simulink model "rudder_Subsystem"  (Simulink 7.8)
settings: Solver=FixedStepDiscrete  SolverMode=SingleTasking  StartTime=0.0  StopTime=10.0  FixedStep=0.01  RelTol=1e-3
InitFcn:
  | clear all
  | common
  | Busses
values from neighbouring files (symbols this model uses):
  T_step = 0.01    [common.m]
undefined symbols (not defined in the file or in its folder): ANmax, CalculateRudderAngle, DataEEInitAndClear, Init_onlyOnce, Init_Reset, initCalibrationRange, InitRudderCalibrationRange, OC1max, RudderCalibrate, RudderEcanInit, RudderSubsystemInit, SendAndReceiveEcan
libraries: dsPICdrivers x17, simulink x4, ecan_dspic x1
settings Model: Creator=bwmairs  LastModifiedBy=Bryant
settings OptimizationCC: InlineParams=on  InlineInvariantSignals=on  InitFltsAndDblsToZero=on  EfficientFloat2IntCast=on
settings DebuggingCC: ReadBeforeWriteMsg=DisableAll  WriteAfterWriteMsg=DisableAll  WriteAfterReadMsg=DisableAll  UnderspecifiedInitializationDetection=Simplified  ParameterOverflowMsg=warning  FcnCallInpInsideContextMsg=Use local settings  UniqueDataStoreMsg=error
settings HardwareCC: ProdBitPerInt=16  ProdBitPerPointer=16  ProdIntDivRoundTo=Zero  ProdEndianess=LittleEndian  ProdWordSize=16  ProdHWDeviceType=16-bit Generic
settings ModelReferenceCC: ModelReferenceNumInstancesAllowed=Single
settings SFSimCC: SimParseCustomCode=off
settings RTWCC: SystemTargetFile=dspic.tlc  GenCodeOnly=on  MakeCommand=make_CreateMPLAB  TemplateMakefile=dspic_pic30_gcc.tmf  PostCodeGenCommand=dsPIC_Compile()  Description=Embedded Target for Microchip dsPIC (real-time)  ProcessScript=dspic_make_rtw_hook  RTWCompilerOptimization=On
settings RTWCC: CustomInclude=|
  | ../../../mavlink/seaslug/sealion
  | ../../../mavlink/seaslug/
  | clib
  | ../basic_model/clib
settings RTWCC: CustomSource=|
  | clib/ecanRudder.c
  | clib/traps.c
  | clib/Nvram.c
  | 
  | ../basic_model/clib/nmea2000.c
  | ../basic_model/clib/DEE.c
  | ../basic_model/clib/DEES.s
  | ../basic_model/clib/MavlinkMessageScheduler.c
  | 
  | ../../../ECAN_dspic/CircularBuffer.c
  | ../../../ECAN_dspic/ecanFunctions.c
settings STFCustomTargetCC: TargetFunctionLibrary=C89/C90 (ANSI)  IncludeMdlTerminateFcn=off  SupportNonInlinedSFcns=off  SystemTargetFile=dspic.tlc
settings ERTTargetCC: TargetFunctionLibrary=C89/C90 (ANSI)  MultiwordLength=2048  ParMdlRefBuildCompliant=off  CompOptLevelCompliant=off  ConcurrentExecutionCompliant=off  IncludeMdlTerminateFcn=off  GeneratePreprocessorConditionals=Disable all  CombineOutputUpdateFcns=off  ERTFirstTimeCompliant=off  ERTCustomFileBanners=off  SupportContinuousTime=on  ModelStepFunctionPrototypeControlCompliant=off  CPPClassGenCompliant=off  ExtModeMexFile=ext_serial_win32_comm  InlinedParameterPlacement=NonHierarchical  ERTSrcFileBannerTemplate=dsPIC_code_template.cgt  ERTHdrFileBannerTemplate=dsPIC_code_template.cgt  ERTDataSrcFileTemplate=dsPIC_code_template.cgt  ERTDataHdrFileTemplate=dsPIC_code_template.cgt  ERTCustomFileTemplate=dsPIC_main.tlc  ConvertIfToSwitch=off  SuppressUnreachableDefaultCases=off
settings CustomProperty: DataType=string  Value=C:\PROGRA~1\MATLAB\R2011b\bin\win64\gmake

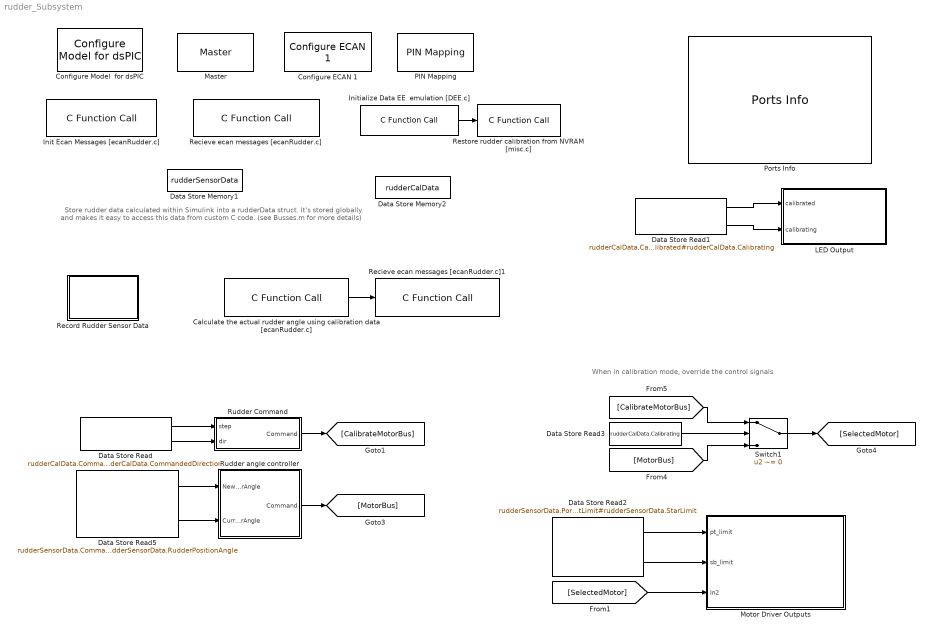
== system rudder_Subsystem ==
  note: When in calibration mode, override the
      | control signals
  note: Store rudder data calculated within Simulink into a rudderData struct.
      | It's stored globally and makes it easy to access this data from custom
      | C code. (see Busses.m for more details)
  Calculate the actual rudder angle using calibration data [ecanRudder.c] : dsPICdrivers/OTHERS/C Function Call  Tag=dsPIC_dsPIC_CFunctionCall  FctUpdate=Output Function  fctName=CalculateRudderAngle  INPUT_SIZE=1  INPUT1=--  INPUT2=--  INPUT3=--  OUTPUT_SIZE=1  OUTPUT1=--  SampleTime=T_step  InputType=[ ]  OutputType=[ ]  FctDeclaration=extern void CalculateRudderAngle();  FctCall=CalculateRudderAngle();  OrderingInOutPopup=Output  FctStart=None  FctStart_Name=Init_onlyOnce  FctStart_Declaration=inline extern void Init_onlyOnce();  FctStart_Call=Init_onlyOnce();  FctInit=None  FctInit_Name=Init_Reset  FctInit_Declaration=inline extern void Init_Reset();  FctInit_Call=Init_Reset();  PinDigitalInput=[]  PinDigitalOutput=[]  AnalogueInput=[]
  Configure ECAN 1 : ecan_dspic/Configure ECAN 1  frame_setting=on  mode=Normal  dma_rx_chan=2  dma_tx_chan=0  baud=250000  ps1=8  pd=5  ps2=6  sjw=4  tq=20  triple_sample=on  dma_buf_size=4 buffers  rx_bufs=[1]  tx_bufs=[0]  buf_0_tx_pri=Highest  buf_0_rte=No  buf_1_tx_pri=Highest  buf_1_rte=No  buf_2_tx_pri=Lowest  buf_2_rte=No  buf_3_tx_pri=Lowest  buf_3_rte=No  buf_4_tx_pri=Lowest  buf_4_rte=No  buf_5_tx_pri=Lowest  buf_5_rte=No  buf_6_tx_pri=Lowest  buf_6_rte=No  buf_7_tx_pri=Lowest  buf_7_rte=No  mask_0=0  mask_0_mide=Match std or ext  mask_1=0  mask_1_mide=Match std or ext  mask_2=0  mask_2_mide=Match std or ext  filters=[0]  filter_0=0  filter_0_mask=0  filter_0_exide=Match only standard  filter_0_buf=1  filter_1=hex2dec('401')  filter_1_mask=0  filter_1_exide=Match only standard  filter_1_buf=2  filter_2=hex2dec('402')  filter_2_mask=0  filter_2_exide=Match only standard  filter_2_buf=3  filter_3=0  filter_3_mask=0  filter_3_exide=Match only standard  filter_3_buf=0  filter_4=0  filter_4_mask=0  filter_4_exide=Match only standard  filter_4_buf=0  filter_5=0  filter_5_mask=0  filter_5_exide=Match only standard  filter_5_buf=0  filter_6=0  filter_6_mask=0  filter_6_exide=Match only standard  filter_6_buf=0  filter_7=0  filter_7_mask=0  filter_7_exide=Match only standard  filter_7_buf=0  filter_8=0  filter_8_mask=0  filter_8_exide=Match only standard  filter_8_buf=0  filter_9=0  filter_9_mask=<empty>  filter_9_exide=Match only standard  filter_9_buf=0  filter_10=0  filter_10_mask=0  filter_10_exide=Match only standard  filter_10_buf=0  filter_11=0  filter_11_mask=0  filter_11_exide=Match only standard  filter_11_buf=0  filter_12=0  filter_12_mask=0  filter_12_exide=Match only standard  filter_12_buf=0  filter_13=0  filter_13_mask=0  filter_13_exide=Match only standard  filter_13_buf=0  filter_14=0  filter_14_mask=0  filter_14_exide=Match only standard  filter_14_buf=0  filter_15=0  filter_15_mask=0  filter_15_exide=Match only standard  filter_15_buf=0
  Configure Model  for dsPIC : dsPICdrivers/Simulink Configuration/Configure Model  for dsPIC
  Data Store Memory1 : DataStoreMemory  DataStoreName=rudderSensorData  ReadBeforeWriteMsg=warning  WriteAfterWriteMsg=warning  WriteAfterReadMsg=warning  OutDataTypeStr=Bus: RudderVariables
      settings: RTWStateStorageClass=ImportedExtern
  Data Store Memory2 : DataStoreMemory  DataStoreName=rudderCalData  ReadBeforeWriteMsg=warning  WriteAfterWriteMsg=warning  WriteAfterReadMsg=warning  OutDataTypeStr=Bus: RudderCalData
      settings: RTWStateStorageClass=ImportedExtern
  Data Store Read : DataStoreRead  DataStoreName=rudderCalData  SampleTime=T_step  DataStoreElements=rudderCalData.CommandedRun#rudderCalData.CommandedDirection
  Data Store Read1 : DataStoreRead  DataStoreName=rudderCalData  SampleTime=T_step  DataStoreElements=rudderCalData.Calibrated#rudderCalData.Calibrating
  Data Store Read2 : DataStoreRead  DataStoreName=rudderSensorData  SampleTime=T_step  DataStoreElements=rudderSensorData.PortLimit#rudderSensorData.StarLimit
  Data Store Read3 : DataStoreRead  DataStoreName=rudderCalData  SampleTime=T_step  DataStoreElements=rudderCalData.Calibrating
  Data Store Read5 : DataStoreRead  DataStoreName=rudderSensorData  SampleTime=T_step  DataStoreElements=rudderSensorData.CommandedRudderAngle#rudderSensorData.RudderPositionAngle
  Init Ecan Messages [ecanRudder.c] : dsPICdrivers/OTHERS/C Function Call  Tag=dsPIC_dsPIC_CFunctionCall  FctUpdate=None  fctName=RudderEcanInit  INPUT_SIZE=1  INPUT1=--  INPUT2=--  INPUT3=--  OUTPUT_SIZE=-1  OUTPUT1=--  SampleTime=Inf  InputType=[]  OutputType=[]  FctDeclaration=extern void RudderEcanInit();  FctCall=RudderEcanInit();  OrderingInOutPopup=None  FctStart=Start Function (Call once and only once)  FctStart_Name=RudderSubsystemInit  FctStart_Declaration=inline extern void RudderSubsystemInit();  FctStart_Call=RudderSubsystemInit();  FctInit=None  FctInit_Name=RudderEcanInit  FctInit_Declaration=inline extern void RudderEcanInit();  FctInit_Call=RudderEcanInit();  PinDigitalInput=[]  PinDigitalOutput=[]  AnalogueInput=[]
  Initialize Data EE  emulation [DEE.c] : dsPICdrivers/OTHERS/C Function Call  Tag=dsPIC_dsPIC_CFunctionCall  FctUpdate=None  fctName='DataEEInitAndClear'  INPUT_SIZE=1  INPUT1=--  INPUT2=--  INPUT3=--  OUTPUT_SIZE=1  OUTPUT1=--  SampleTime=Inf  InputType=[]  OutputType=[]  FctDeclaration=extern void DataEEInitAndClear();  FctCall=DataEEInitAndClear();  OrderingInOutPopup=Output  FctStart=Start Function (Call once and only once)  FctStart_Name=DataEEInitAndClear  FctStart_Declaration=inline extern void DataEEInitAndClear();  FctStart_Call=DataEEInitAndClear();  FctInit=None  FctInit_Name=Init_Reset  FctInit_Declaration=inline extern void Init_Reset();  FctInit_Call=Init_Reset();  PinDigitalInput=[]  PinDigitalOutput=[]  AnalogueInput=[]
  LED Output : Subsystem
  Master : dsPICdrivers/Master  Tag=dsPIC_MASTER  Priority=1  TimeStepType=Timer1  picType=33fj128MC802  fcy=40008571.4286  Quartz_33f=8e6  PLLActive_33f=on  fcyDesired_33f=40000000  tmr1="[8  50010  -0.00057131]"  tmr1Info="Time Step : 0.01  ;   Error : -0.00057131%  PR1=50010"  tmr2345="[8  0  0  0]"  tmr2345cfg=[-1 -1 -1 -1]  IOautoConf=on  typePort="[ 9   8   0   0  10   0   0   0   0   0   0   0   0   0   0   0   0   9   8   0  22   0   0  23   0  10  10   0  23   0   0   0   0   0   0   0   0   0   0   0   0   0   0   0   0   0   0   0   0   0   0   0   0   0   0   0   0   0   0   0   0   0   0   0   0   0   0   0   0   0   0   0   0   0   0   0   0   0   0   0   0   0   0   0   0   0   0   0   0   0   0   0   0   0   0   0   0   0   0   0   0   0   0   0   0   0   0   0   0   0   0   0 ]"  TRIS="[ 65519  59775  65535  65535  65535  65535  65535 ]"  ADPCFG=9  MasterBusyPort=None  MasterOverloadPort=None  FOSC=Internal Fast RC 7.37Mhz  ClockSwitchMonitor=Both disabled  TempProtection_33f=TEMP_ON  FPBOR=<empty>  PWRT=disable  MCLR=<empty>  ICD=ICS_PGD3  JTAGEN=JTAGEN_OFF  PowerSave=off  OverrideFcy=off  NewFcy=1e6  PR2345="[65535  65535  65535  65535]"
  Motor Driver Outputs : Subsystem
  PIN Mapping : dsPICdrivers/Peripheral MAPPING/PIN Mapping  Tag=dsPIC_PIN_Mapping  in_INT1=Not tied (VSS)  in_INT2=Not tied (VSS)  in_T2CK=Not tied (VSS)  in_T3CK=Not tied (VSS)  in_T4CK=Not tied (VSS)  in_T5CK=Not tied (VSS)  in_IC1=Not tied (VSS)  in_IC2=Not tied (VSS)  in_IC7=Not tied (VSS)  in_IC8=Not tied (VSS)  out_OC1=tied to RP12  out_OC2=Not changed  out_OC3=Not changed  out_OC4=Not changed  in_OCFA=Not tied (VSS)  in_FLTA1=Not tied (VSS)  in_FLTA2=Not tied (VSS)  in_QEA1=Not tied (VSS)  in_QEB1=Not tied (VSS)  in_INDX1=Not tied (VSS)  out_UPDN1=Not changed  out_UPDN2=Not changed  in_QEA2=Not tied (VSS)  in_QEB2=Not tied (VSS)  in_INDX2=Not tied (VSS)  in_U1RX=Not tied (VSS)  out_U1TX=Not changed  in_U1CTS=Not tied (VSS)  out_U1RTS=Not changed  in_U2RX=Not tied (VSS)  out_U2TX=Not changed  in_U2CTS=Not tied (VSS)  out_U2RTS=Not changed  in_SDI1=Not tied (VSS)  out_SDO1=Not changed  in_SCK1=Not tied (VSS)  out_SCK1OUT=Not changed  in_SS1=Not tied (VSS)  out_SS1OUT=Not changed  in_SDI2=Not tied (VSS)  out_SDO2=Not changed  in_SCK2=Not tied (VSS)  out_SCK2OUT=Not changed  in_SS2=Not tied (VSS)  out_SS2OUT=Not changed  in_C1RX=tied to RP4  out_C1TX=tied to RP7  out_C1OUT=Not changed  out_C2OUT=Not changed
  Ports Info : dsPICdrivers/Ports Info  Tag=dsPIC_PortInfo
  Recieve ecan messages [ecanRudder.c] : dsPICdrivers/OTHERS/C Function Call  Tag=dsPIC_dsPIC_CFunctionCall  FctUpdate=Output Function  fctName=SendAndReceiveEcan  INPUT_SIZE=1  INPUT1=--  INPUT2=--  INPUT3=--  OUTPUT_SIZE=1  OUTPUT1=--  SampleTime=.01  InputType=[ ]  OutputType=[ ]  FctDeclaration=extern void SendAndReceiveEcan();  FctCall=SendAndReceiveEcan();  OrderingInOutPopup=None  FctStart=None  FctStart_Name=Init_onlyOnce  FctStart_Declaration=inline extern void Init_onlyOnce();  FctStart_Call=Init_onlyOnce();  FctInit=None  FctInit_Name=Init_Reset  FctInit_Declaration=inline extern void Init_Reset();  FctInit_Call=Init_Reset();  PinDigitalInput=[]  PinDigitalOutput=[]  AnalogueInput=[]
  Recieve ecan messages [ecanRudder.c]1 : dsPICdrivers/OTHERS/C Function Call  Tag=dsPIC_dsPIC_CFunctionCall  FctUpdate=Output Function  fctName=RudderCalibrate  INPUT_SIZE=1  INPUT1=--  INPUT2=--  INPUT3=--  OUTPUT_SIZE=1  OUTPUT1=--  SampleTime=T_step  InputType=[ ]  OutputType=[ ]  FctDeclaration=extern void RudderCalibrate();  FctCall=RudderCalibrate();  OrderingInOutPopup=Input  FctStart=None  FctStart_Name=Init_onlyOnce  FctStart_Declaration=inline extern void Init_onlyOnce();  FctStart_Call=Init_onlyOnce();  FctInit=None  FctInit_Name=Init_Reset  FctInit_Declaration=inline extern void Init_Reset();  FctInit_Call=Init_Reset();  PinDigitalInput=[]  PinDigitalOutput=[]  AnalogueInput=[]
  Record Rudder Sensor Data : Subsystem
  Restore rudder calibration from NVRAM [misc.c] : dsPICdrivers/OTHERS/C Function Call  Tag=dsPIC_dsPIC_CFunctionCall  FctUpdate=None  fctName='initCalibrationRange'  INPUT_SIZE=1  INPUT1=--  INPUT2=--  INPUT3=--  OUTPUT_SIZE=1  OUTPUT1=--  SampleTime=Inf  InputType=[]  OutputType=[]  FctDeclaration=extern void initCalibrationRange();  FctCall=initCalibrationRange();  OrderingInOutPopup=Input  FctStart=Start Function (Call once and only once)  FctStart_Name=InitRudderCalibrationRange  FctStart_Declaration=inline extern void InitRudderCalibrationRange();  FctStart_Call=InitRudderCalibrationRange();  FctInit=None  FctInit_Name=Init_Reset  FctInit_Declaration=inline extern void Init_Reset();  FctInit_Call=Init_Reset();  PinDigitalInput=[]  PinDigitalOutput=[]  AnalogueInput=[]
  Rudder Command : Subsystem
  Rudder angle controller : Subsystem
  Switch1 : Switch  Criteria=u2 ~= 0
  wires:
  Data Store Read/1 -> Rudder Command/1(step)
  Data Store Read/2 -> Rudder Command/2(dir)
  Rudder Command/1(Command) -> [CalibrateMotorBus]
  [SelectedMotor] -> Motor Driver Outputs/3(In2)
  Rudder angle controller/1(Command) -> [MotorBus]
  [CalibrateMotorBus] -> Switch1/1
  [MotorBus] -> Switch1/3
  Switch1/1 -> [SelectedMotor]
  Data Store Read5/2 -> Rudder angle controller/2(CurrentRudderAngle)
  Data Store Read5/1 -> Rudder angle controller/1(NewRudderAngle)
  Initialize Data EE  emulation [DEE.c]/1 -> Restore rudder calibration from NVRAM [misc.c]/1
  Calculate the actual rudder angle using calibration data [ecanRudder.c]/1 -> Recieve ecan messages [ecanRudder.c]1/1
  Data Store Read1/1 -> LED Output/1(calibrated)
  Data Store Read1/2 -> LED Output/2(calibrating)
  Data Store Read2/1 -> Motor Driver Outputs/1(pt_limit)
  Data Store Read2/2 -> Motor Driver Outputs/2(sb_limit)
  Data Store Read3/1 -> Switch1/2

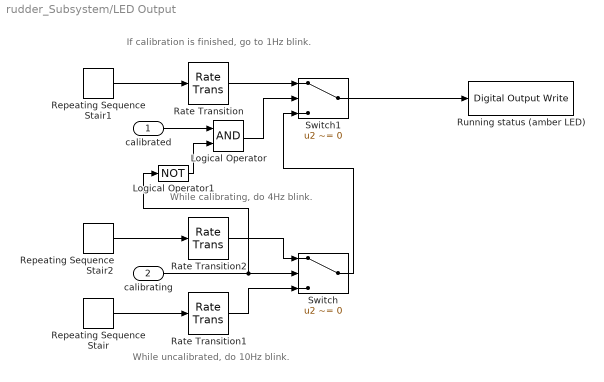
== system rudder_Subsystem/LED Output ==
  note: If calibration is finished, go to 1Hz blink.
  note: While calibrating, do 4Hz blink.
  note: While uncalibrated, do 10Hz blink.
  calibrated : Inport
  calibrating : Inport  Port=2
  Logical Operator : Logic  AllPortsSameDT=off  OutDataTypeStr=boolean
  Logical Operator1 : Logic  Operator=NOT  AllPortsSameDT=off  OutDataTypeStr=boolean
  Rate Transition : RateTransition
  Rate Transition1 : RateTransition
  Rate Transition2 : RateTransition
  Repeating Sequence Stair : simulink/Sources/Repeating Sequence Stair  OutValues=[1 0]  tsamp=.1  OutMin=[]  OutMax=[]  OutDataTypeStr=fixdt('boolean')  OutputDataTypeScalingMode=Specify via dialog  OutDataType=fixdt('boolean')  ConRadixGroup=Best Precision: Vector-wise  OutScaling=[]
  Repeating Sequence Stair1 : simulink/Sources/Repeating Sequence Stair  OutValues=[1 0]  tsamp=1  OutMin=[]  OutMax=[]  OutDataTypeStr=fixdt('boolean')  OutputDataTypeScalingMode=Specify via dialog  OutDataType=fixdt('boolean')  ConRadixGroup=Best Precision: Vector-wise  OutScaling=[]
  Repeating Sequence Stair2 : simulink/Sources/Repeating Sequence Stair  OutValues=[1 0]  tsamp=.25  OutMin=[]  OutMax=[]  OutDataTypeStr=fixdt('boolean')  OutputDataTypeScalingMode=Specify via dialog  OutDataType=fixdt('boolean')  ConRadixGroup=Best Precision: Vector-wise  OutScaling=[]
  Running status (amber LED) : dsPICdrivers/Digital I//O/Digital Output Write  Tag=dsPIC_Digital_Output  Priority=5  PORT=A  Pin=[4]  Simultaneous=off  OrderingInOutPopup=None
  Switch : Switch  Criteria=u2 ~= 0
  Switch1 : Switch  Criteria=u2 ~= 0
  wires:
  Repeating Sequence Stair/1 -> Rate Transition1/1
  Rate Transition1/1 -> Switch/3
  calibrating/1 -> Switch/2, Logical Operator1/1
  Repeating Sequence Stair1/1 -> Rate Transition/1
  Rate Transition/1 -> Switch1/1
  Repeating Sequence Stair2/1 -> Rate Transition2/1
  Rate Transition2/1 -> Switch/1
  Switch1/1 -> Running status (amber LED)/1
  Switch/1 -> Switch1/3
  calibrated/1 -> Logical Operator/1
  Logical Operator/1 -> Switch1/2
  Logical Operator1/1 -> Logical Operator/2

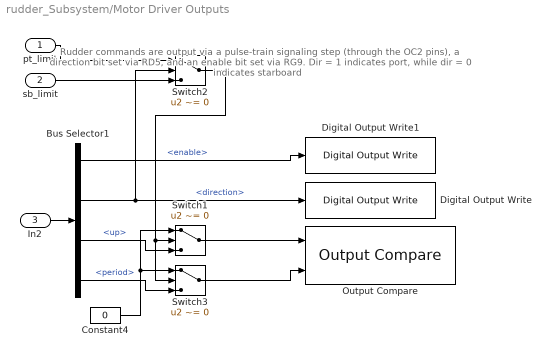
== system rudder_Subsystem/Motor Driver Outputs ==
  note: Rudder commands are output via a pulse-train signaling step (through the OC2 pins),
      | a direction bit set via RD5, and an enable bit set via RG9. Dir = 1 indicates port, while
      | dir = 0 indicates starboard
  pt_limit : Inport
  sb_limit : Inport  Port=2
  In2 : Inport  Port=3
  Bus Selector1 : BusSelector  OutputSignals=enable,direction,up,period
  Constant4 : Constant  Value=0  OutDataTypeStr=uint16
  Digital Output Write : dsPICdrivers/Digital I//O/Digital Output Write  Tag=dsPIC_Digital_Output  Priority=5  PORT=B  Pin=[9]  Simultaneous=off  OrderingInOutPopup=None
  Digital Output Write1 : dsPICdrivers/Digital I//O/Digital Output Write  Tag=dsPIC_Digital_Output  Priority=5  PORT=B  Pin=[10]  Simultaneous=off  OrderingInOutPopup=None
  Output Compare : dsPICdrivers/Peripheral I//O/Output Compare  Tag=dsPIC_PWM_out  Priority=5  IntPriority=3  CHANNEL=[1]  Channel_UP_Down_Periode=[5]  MaxChannel=[0.01]  MaxName=' OC1max '  Precision=[15.6099]  Timer=[2]  Status=OK  SafeMarge=[0]  PortLetter=[66]  PortNumber=[12]  MaxValues=[50010]
  Switch1 : Switch  Criteria=u2 ~= 0  Threshold=1  OutDataTypeStr=Inherit: Inherit via back propagation
  Switch2 : Switch  Criteria=u2 ~= 0  Threshold=1  OutDataTypeStr=Inherit: Inherit via back propagation
  Switch3 : Switch  Criteria=u2 ~= 0  Threshold=1  OutDataTypeStr=Inherit: Inherit via back propagation
  wires:
  Bus Selector1/1 -> Digital Output Write1/1  "<enable>"
  Switch2/1 -> Switch1/2, Switch3/2
  Constant4/1 -> Switch1/1, Switch3/1
  Bus Selector1/4 -> Switch3/3  "<period>"
  Bus Selector1/3 -> Switch1/3  "<up>"
  Switch1/1 -> Output Compare/1
  Switch3/1 -> Output Compare/2
  Bus Selector1/2 -> Digital Output Write/1, Switch2/2  "<direction>"
  pt_limit/1 -> Switch2/1
  In2/1 -> Bus Selector1/1
  sb_limit/1 -> Switch2/3

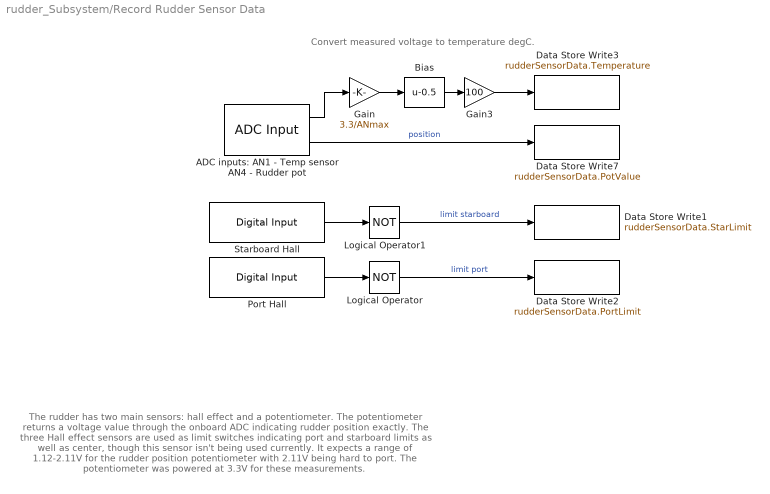
== system rudder_Subsystem/Record Rudder Sensor Data ==
  note: The rudder has two main sensors: hall effect and a potentiometer. The
      | potentiometer returns a voltage value through the onboard ADC indicating
      | rudder position exactly. The three Hall effect sensors are used as limit switches
      | indicating port and starboard limits as well as center, though this sensor isn't
      | being used currently.
      |
      | It expects a range of 1.12-2.11V for the rudder position potentiometer with
      | 2.11V being hard to port. The potentiometer was powered at 3.3V for these
      | measurements.
  note: Convert measured voltage to temperature degC.
  ADC inputs: AN1 - Temp sensor AN4 - Rudder pot : dsPICdrivers/Peripheral I//O/ADC Input  Tag=dsPIC_ADC  Priority=5  ADC_TYPE=12 bits  ADC_MODE=Continuous sampling & get last channel value  NbrSampleStep=1  VoltRefpopup="AVdd  -  AVss"  OutFormatBitspopup=0000 dddd dddd dddd : Integer  InterruptPriority=6  ANCHANNELS=[4 1]  MaxName=ANmax = 4095  Rin=0  ADCS=53  SAMC=1  Temperature=25  DMAChannel=1  SampleTime=T_step  Status="OK  |  Tsmp=6.749e-007 |  T/Channel=1.012e-005 |  Tall=2.025e-005"  SSRC=auto convert
  Bias : Bias  Bias=-0.5
  Data Store Write1 : DataStoreWrite  DataStoreName=rudderSensorData  DataStoreElements=rudderSensorData.StarLimit
  Data Store Write2 : DataStoreWrite  DataStoreName=rudderSensorData  DataStoreElements=rudderSensorData.PortLimit
  Data Store Write3 : DataStoreWrite  DataStoreName=rudderSensorData  DataStoreElements=rudderSensorData.Temperature
  Data Store Write7 : DataStoreWrite  DataStoreName=rudderSensorData  DataStoreElements=rudderSensorData.PotValue
  Gain : Gain  Gain=3.3/ANmax  ParamDataTypeStr=single  OutDataTypeStr=single  RndMeth=Simplest
  Gain3 : Gain  Gain=100  ParamDataTypeStr=single  OutDataTypeStr=single  RndMeth=Simplest
  Logical Operator : Logic  Operator=NOT  Inputs=1  AllPortsSameDT=off  OutDataTypeStr=boolean
  Logical Operator1 : Logic  Operator=NOT  Inputs=1  AllPortsSameDT=off  OutDataTypeStr=boolean
  Port Hall : dsPICdrivers/Digital I//O/Digital Input  Tag=dsPIC_Digital_Input  PORT=A  Pin=[0]  SampleTime=T_step  OrderingInOutPopup=None
  Starboard Hall : dsPICdrivers/Digital I//O/Digital Input  Tag=dsPIC_Digital_Input  PORT=B  Pin=[1]  SampleTime=T_step  OrderingInOutPopup=None
  wires:
  Logical Operator1/1 -> Data Store Write1/1  "limit starboard"
  Logical Operator/1 -> Data Store Write2/1  "limit port"
  Port Hall/1 -> Logical Operator/1
  Starboard Hall/1 -> Logical Operator1/1
  ADC inputs: AN1 - Temp sensor AN4 - Rudder pot/2 -> Data Store Write7/1  "position"
  ADC inputs: AN1 - Temp sensor AN4 - Rudder pot/1 -> Gain/1
  Gain/1 -> Bias/1
  Bias/1 -> Gain3/1
  Gain3/1 -> Data Store Write3/1

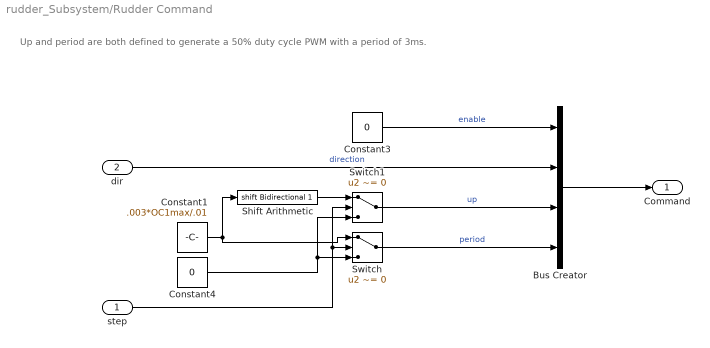
== system rudder_Subsystem/Rudder Command ==
  note: Up and period are both defined to generate a 50% duty cycle PWM with
      | a period of 3ms.
  step : Inport
  dir : Inport  Port=2
  Bus Creator : BusCreator
  Constant1 : Constant  Value=.003*OC1max/.01  OutDataTypeStr=uint16
  Constant3 : Constant  Value=0  OutDataTypeStr=boolean
  Constant4 : Constant  Value=0  OutDataTypeStr=uint16
  Shift Arithmetic : ArithShift  BitShiftNumber=1
  Switch : Switch  Criteria=u2 ~= 0
  Switch1 : Switch  Criteria=u2 ~= 0
  Command : Outport
  wires:
  step/1 -> Switch1/2, Switch/2
  Constant4/1 -> Switch1/3, Switch/3
  Switch1/1 -> Bus Creator/3  "up"
  Switch/1 -> Bus Creator/4  "period"
  Shift Arithmetic/1 -> Switch1/1
  Constant1/1 -> Switch/1, Shift Arithmetic/1
  Constant3/1 -> Bus Creator/1  "enable"
  Bus Creator/1 -> Command/1
  dir/1 -> Bus Creator/2  "direction"

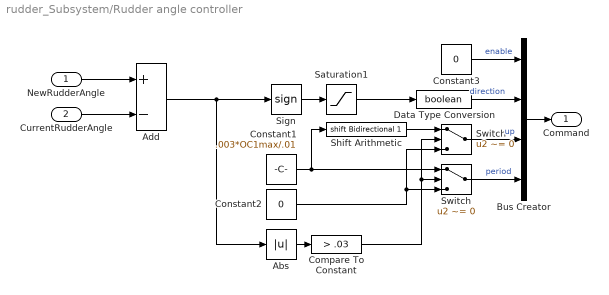
== system rudder_Subsystem/Rudder angle controller ==
  NewRudderAngle : Inport
  CurrentRudderAngle : Inport  Port=2
  Abs : Abs
  Add : Sum  Inputs=+-
  Bus Creator : BusCreator
  Compare To Constant : simulink/Logic and Bit Operations/Compare To Constant  relop=>  const=.03  OutDataTypeStr=boolean
  Constant1 : Constant  Value=.003*OC1max/.01  OutDataTypeStr=uint16
  Constant2 : Constant  Value=0  OutDataTypeStr=uint16
  Constant3 : Constant  Value=0  OutDataTypeStr=boolean
  Data Type Conversion : DataTypeConversion  OutDataTypeStr=boolean  RndMeth=Simplest
  Saturation1 : Saturate  UpperLimit=1  LowerLimit=0  OutDataTypeStr=Inherit: Inherit via back propagation
  Shift Arithmetic : ArithShift  BitShiftNumber=1
  Sign : Signum
  Switch : Switch  Criteria=u2 ~= 0
  Switch4 : Switch  Criteria=u2 ~= 0
  Command : Outport
  wires:
  Add/1 -> Abs/1, Sign/1
  Compare To Constant/1 -> Switch4/2, Switch/2
  Constant2/1 -> Switch4/3, Switch/3
  Switch4/1 -> Bus Creator/3  "up"
  Switch/1 -> Bus Creator/4  "period"
  Shift Arithmetic/1 -> Switch4/1
  Abs/1 -> Compare To Constant/1
  Constant1/1 -> Switch/1, Shift Arithmetic/1
  Constant3/1 -> Bus Creator/1  "enable"
  Sign/1 -> Saturation1/1
  Saturation1/1 -> Data Type Conversion/1
  Data Type Conversion/1 -> Bus Creator/2  "direction"
  NewRudderAngle/1 -> Add/1
  Bus Creator/1 -> Command/1
  CurrentRudderAngle/1 -> Add/2
